simulink model "untitled2"  (Simulink 7.9)
settings: Solver=FixedStepDiscrete  StartTime=0.0  StopTime=1/48000  FixedStep=1/48000  RelTol=1e-3
undefined symbols (not defined in the file or in its folder): j
libraries: dspxfrm3 x1
settings Model: Creator=Estilo  LastModifiedBy=Estilo

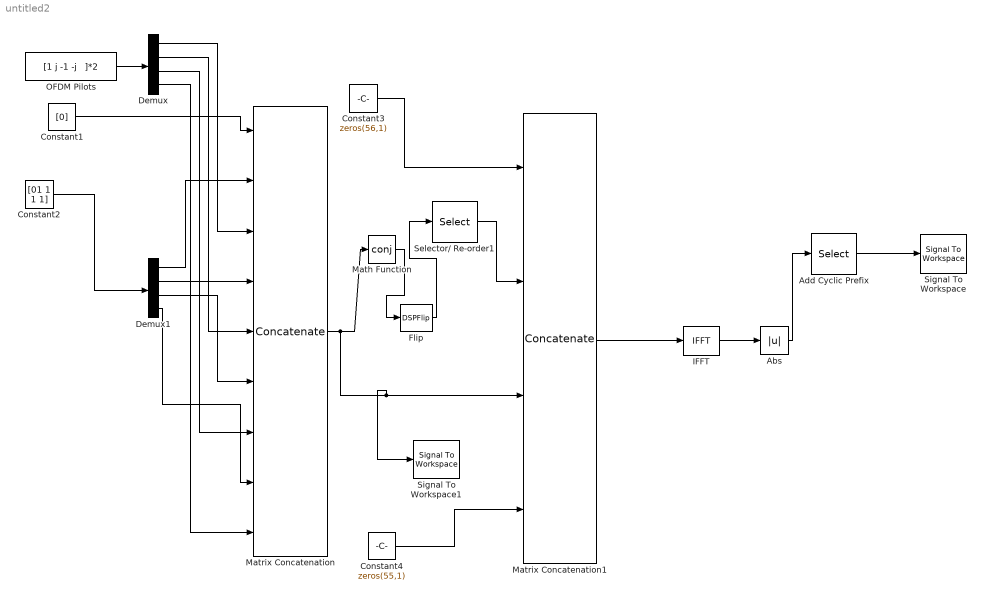
== system untitled2 ==
  Abs : Abs
  Add Cyclic Prefix : Selector  InputPortWidth=128  IndexOptions=Index vector (dialog)  Indices=[97:128 1:128]  OutputSizes=1
  Constant1 : Constant  Value=[0]
  Constant2 : Constant  Value=[01 1 1 1]
  Constant3 : Constant  Value=zeros(56,1)
  Constant4 : Constant  Value=zeros(55,1)
  Demux : Demux
  Demux1 : Demux
  Flip : DSPFlip
  IFFT : dspxfrm3/IFFT  CompMethod=Table lookup  TableOpt=HYBRID  TableOptActive=Speed  BitRevOrder=off  cs_in=off  SkipNorm=on  InheritFFTLength=on  FFTLength=64  mode=Complex  outSamplingMode=Frame based  RowConvenienceOn=on  FFTImplementation=Auto  firstCoeffDataTypeStr=Inherit: Same word length as input  firstCoeffLastDataTypeStr=Inherit: Same word length as input  outputMin=[]  outputMax=[]  roundingMode=Floor  overflowMode=off
  Math Function : Math  Operator=conj  SaturateOnIntegerOverflow=on
  Matrix Concatenation : Concatenate  NumInputs=9  Mode=Multidimensional array
  Matrix Concatenation1 : Concatenate  NumInputs=4  Mode=Multidimensional array
  OFDM Pilots : Constant  Value="[1 j -1 -j   ]*2"
  Selector/ Re-order1 : Selector  InputPortWidth=9  IndexOptions=Index vector (dialog)  Indices=[1:8]  OutputSizes=1
  Signal To Workspace : SignalToWorkspace  VariableName=yout1
      settings: CopyFcn=dspblkcopystw(gcbh);
  Signal To Workspace1 : SignalToWorkspace  VariableName=yout
      settings: CopyFcn=dspblkcopystw(gcbh);
  wires:
  Constant1/1 -> Matrix Concatenation/1
  Demux1/4 -> Matrix Concatenation/8
  Demux1/3 -> Matrix Concatenation/6
  Demux1/2 -> Matrix Concatenation/4
  Demux1/1 -> Matrix Concatenation/2
  Constant2/1 -> Demux1/1
  OFDM Pilots/1 -> Demux/1
  Demux/1 -> Matrix Concatenation/3
  Demux/2 -> Matrix Concatenation/5
  Demux/3 -> Matrix Concatenation/7
  Demux/4 -> Matrix Concatenation/9
  Constant3/1 -> Matrix Concatenation1/1
  Matrix Concatenation/1 -> Math Function/1, Matrix Concatenation1/3, Signal To Workspace1/1
  Math Function/1 -> Flip/1
  Flip/1 -> Selector/ Re-order1/1
  Selector/ Re-order1/1 -> Matrix Concatenation1/2
  Constant4/1 -> Matrix Concatenation1/4
  Matrix Concatenation1/1 -> IFFT/1
  IFFT/1 -> Abs/1
  Abs/1 -> Add Cyclic Prefix/1
  Add Cyclic Prefix/1 -> Signal To Workspace/1
